simulink model "copyofXiongyun"  (R2024a)
settings: Solver=VariableStepAuto  StartTime=0.0  StopTime=0.0009216  RelTol=1e-3
model workspace (MAT data in the model file):
  Delay_64 = [8.33333333333e-08 8.33333333334e-08 8.33333333334e-08]
  ENOB_64 = 9.79993802046
  FUNDF_64 = [976365.653838 1576901.29512]
  FUNDX_64 = [80.1059011122 2.28890713222]
  IMODF_64 = [354414.165404 2174124.62014]
  IMODX_64 = [-0.261373749224 0.226791798058]
  NoiseFloor_64 = -9.93722436924
  OIP3_64 = 61.8047516711
  SFDR_64 = 80.4342870842
  SINAD_64 = 60.7556268832
  SNR_64 = 60.8263157789
  THD_64 = -76.0066685253
  delay_64 = [8.33333333333e-08 8.33333333334e-08 8.33333333334e-08]
libraries: msbAdcMeasurements x1, dspsigops x1
settings Model: Creator=sjtu  LastModifiedBy=sjtu
settings DebuggingCC: SFUnexpectedBacktrackingDiag=warning

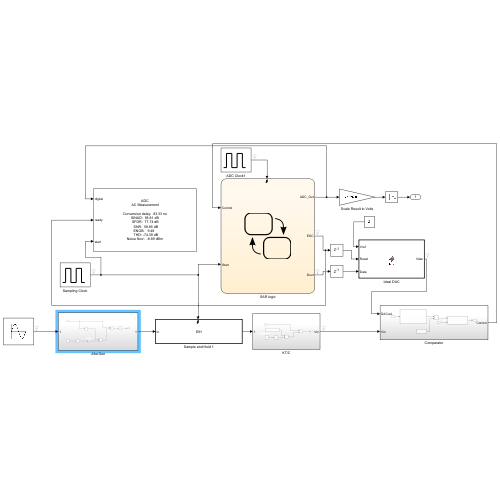
[thumbnail: Simulink's stored preview of the top-level diagram]
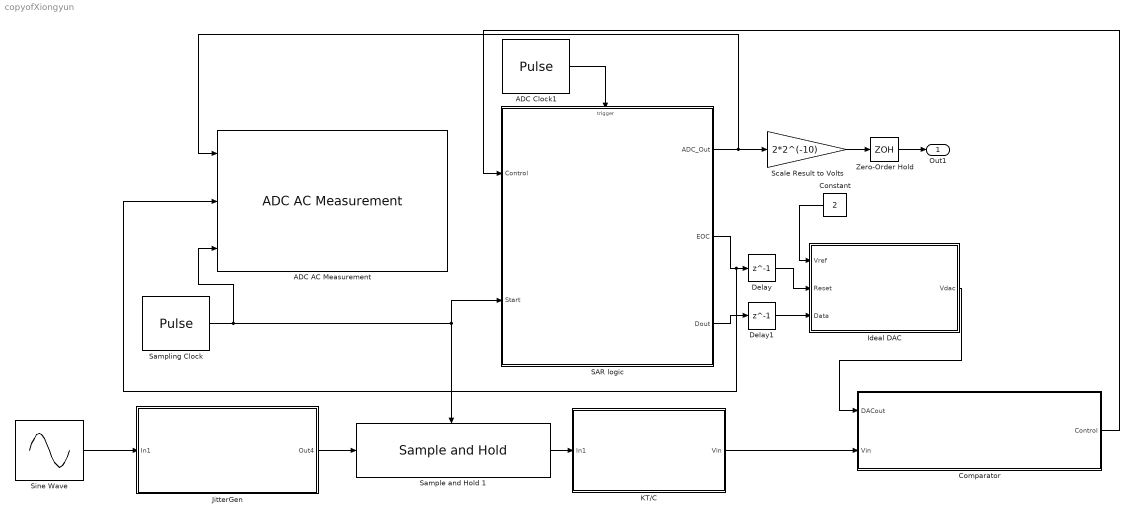
== system copyofXiongyun ==
  ADC AC Measurement : msbAdcMeasurements/ADC AC Measurement  DistortionMeasurement=Harmonic  InputFrequency=9.729e5  Method=Filter bank (slower, more precise, low leakage)  RBW=9765.625  AutoSetRBW=on  NBits=5  Frequency=1e7  HoldOffTime=0  OutputToWorkspace=off  VariableName=adc_ac_out  ShowSpectrum=off
      link override ADC AC Measurement/ADC AC Measurement Spectrum Analyzer: YLimits=[-95.22924158514904,96.56585219838266]  SpectrumUnits=Auto  FrequencyScale=Log  ViewType=Spectrum
  ADC Clock1 : DiscretePulseGenerator  PulseType=Time based  Period=100e-9/12  PulseWidth=50
  Comparator : Subsystem
  Constant : Constant  Value=2
  Delay : Delay  DelayLength=1  InitialCondition=0
  Delay1 : Delay  DelayLength=1  InitialCondition=0
  Ideal DAC : MATLAB Function  TreatAsAtomicUnit=on
  JitterGen : Subsystem
  KT/C : Subsystem
  SAR logic : Stateflow chart  TreatAsAtomicUnit=on
  Sample and Hold 1 : dspsigops/Sample and Hold  trig=Rising edge  initCond=0  latchinput=off
  Sampling Clock : DiscretePulseGenerator  PulseType=Time based  Period=100e-9  PulseWidth=50  PhaseDelay=50e-9
  Scale Result to Volts : Gain  Gain=2*2^(-10)  ParamDataTypeStr=double  OutDataTypeStr=double
  Sine Wave : Sin  Frequency=2*pi*9.729e5  SampleTime=0
  Zero-Order Hold : ZeroOrderHold  SampleTime=-1
  Out1 : Outport
  wires:
  Sampling Clock/1 -> ADC AC Measurement/3, Sample and Hold 1/Trigger, SAR logic/2(Start)
  Sine Wave/1 -> JitterGen/1(In1)
  JitterGen/1(Out4) -> Sample and Hold 1/1
  Sample and Hold 1/1 -> KT/C/1(In1)
  KT/C/1(Vin) -> Comparator/2(Vin)
  ADC Clock1/1 -> SAR logic/Trigger
  Ideal DAC/1(Vdac) -> Comparator/1(DACout)
  Comparator/1(Control) -> SAR logic/1(Control)
  Constant/1 -> Ideal DAC/1(Vref)
  SAR logic/1(ADC_Out) -> ADC AC Measurement/1, Scale Result to Volts/1
  Scale Result to Volts/1 -> Zero-Order Hold/1
  Zero-Order Hold/1 -> Out1/1
  Delay/1 -> Ideal DAC/2(Reset)
  SAR logic/3(Dout) -> Delay1/1
  Delay1/1 -> Ideal DAC/3(Data)
  SAR logic/2(EOC) -> ADC AC Measurement/2, Delay/1

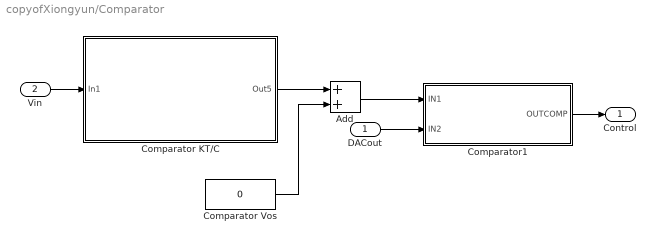
== system copyofXiongyun/Comparator ==
  DACout : Inport
  Vin : Inport  Port=2
  Add : Sum
  Comparator KT/C : Subsystem
  Comparator Vos : Constant  Value=0
  Comparator1 : MATLAB Function  TreatAsAtomicUnit=on
  Control : Outport
  wires:
  Comparator1/1(OUTCOMP) -> Control/1
  Vin/1 -> Comparator KT/C/1(In1)
  Comparator KT/C/1(Out5) -> Add/1
  Add/1 -> Comparator1/1(IN1)
  Comparator Vos/1 -> Add/2
  DACout/1 -> Comparator1/2(IN2)

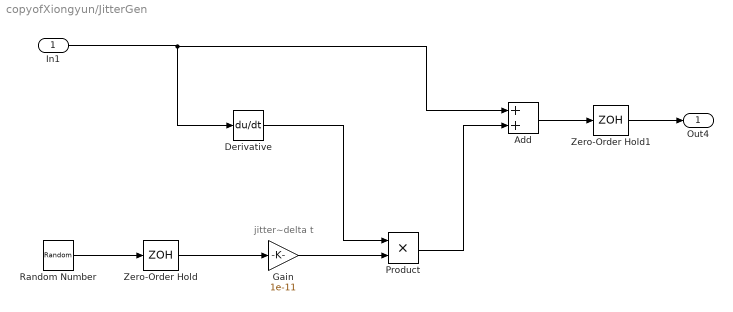
== system copyofXiongyun/JitterGen ==
  note: jitter~delta t
  In1 : Inport
  Add : Sum
  Derivative : Derivative
  Gain : Gain  Gain=1e-11
  Product : Product
  Random Number : RandomNumber  SampleTime=1e-9
  Zero-Order Hold : ZeroOrderHold  SampleTime=-1
  Zero-Order Hold1 : ZeroOrderHold  SampleTime=-1
  Out4 : Outport
  wires:
  Gain/1 -> Product/2
  Random Number/1 -> Zero-Order Hold/1
  Product/1 -> Add/2
  In1/1 -> Add/1, Derivative/1
  Zero-Order Hold/1 -> Gain/1
  Add/1 -> Zero-Order Hold1/1
  Derivative/1 -> Product/1
  Zero-Order Hold1/1 -> Out4/1

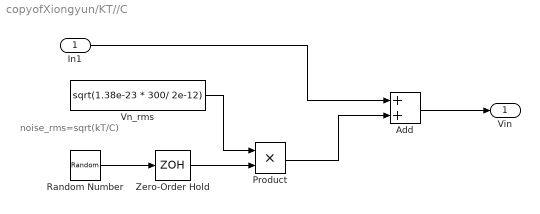
== system copyofXiongyun/KT//C ==
  note: noise_rms=sqrt(kT/C)
  In1 : Inport
  Add : Sum
  Product : Product
  Random Number : RandomNumber  SampleTime=1e-9
  Vn_rms : Constant  Value=sqrt(1.38e-23 * 300/ 2e-12)
  Zero-Order Hold : ZeroOrderHold  SampleTime=-1
  Vin : Outport
  wires:
  Vn_rms/1 -> Product/1
  In1/1 -> Add/1
  Random Number/1 -> Zero-Order Hold/1
  Zero-Order Hold/1 -> Product/2
  Add/1 -> Vin/1
  Product/1 -> Add/2

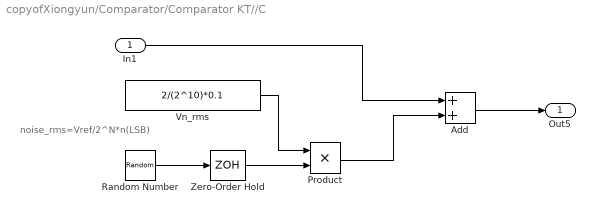
== system copyofXiongyun/Comparator/Comparator KT//C ==
  note: noise_rms=Vref/2^N*n(LSB)
  In1 : Inport
  Add : Sum
  Product : Product
  Random Number : RandomNumber  SampleTime=1e-9
  Vn_rms : Constant  Value=2/(2^10)*0.1
  Zero-Order Hold : ZeroOrderHold  SampleTime=-1
  Out5 : Outport
  wires:
  Vn_rms/1 -> Product/1
  In1/1 -> Add/1
  Random Number/1 -> Zero-Order Hold/1
  Zero-Order Hold/1 -> Product/2
  Add/1 -> Out5/1
  Product/1 -> Add/2

== matlab function copyofXiongyun/Ideal DAC ==
  data: Vref input; Reset input; Data input; Vdac output
function Vdac = fcn(Vref,Reset,Data)
if Reset==1
    Vdac=0;
else
    Vdac=double(Data)*Vref/(2^10);
end

== matlab function copyofXiongyun/Comparator/Comparator1 ==
  data: IN1 input; OUTCOMP output; IN2 input
function OUTCOMP = fcn(IN1,IN2)
if IN1>=IN2
    OUTCOMP=1;
else
    OUTCOMP=0;
end

== stateflow chart copyofXiongyun/SAR logic ==
  settings: executeAtInitialization=1
  state Idle_Done
    entry: Bit=9;
    EOC=1;
    ADC_Out=Dout;
  state Run
    entry: Dout=Dout+2^Bit;
  (default) -> Idle_Done
  (junction 26) -> Idle_Done [order 2] : [Bit==0]
  Idle_Done -> Run : [Start==1]{Dout=-2^Bit;EOC=0;}
  (junction 26) -> Run [order 1] : [Bit>0]{Bit=Bit-1;}
  Run -> (junction 7) [order 2] : [Control==1]
  Run -> (junction 7) [order 1] : [Control==0]{Dout=Dout-2^Bit;}
  (junction 7) -> (junction 26)
  data: Control input; Start input; ADC_Out output int16; EOC output; Bit local double =9; Dout output int16
  events: clk input RISING_EDGE_EVENT
